simulink model "rsa_simulink"  (R2015a)
settings: Solver=ode45  StartTime=0.0  StopTime=1  RelTol=1e-3
settings Model: Creator=Hp  LastModifiedBy=Hp

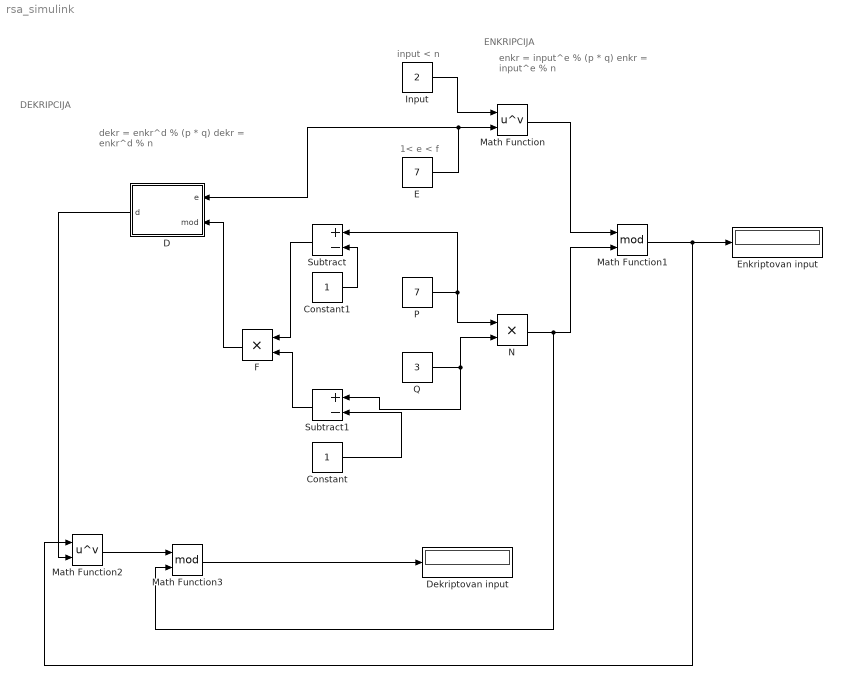
== system rsa_simulink ==
  note: 1< e < f
  note: ENKRIPCIJA
  note: DEKRIPCIJA
  note: enkr = input^e % (p * q)
      | enkr = input^e % n
  note: dekr = enkr^d % (p * q)
      | dekr = enkr^d % n
  note: input < n
  Constant : Constant
  Constant1 : Constant
  D : MATLAB Function  TreatAsAtomicUnit=on
  Dekriptovan input : Display
  E : Constant  Value=7
  Enkriptovan input : Display
  "F " : Product
  Input : Constant  Value=2
  Math Function : Math  Operator=pow  SaturateOnIntegerOverflow=on
  Math Function1 : Math  Operator=mod  SaturateOnIntegerOverflow=on
  Math Function2 : Math  Operator=pow  SaturateOnIntegerOverflow=on
  Math Function3 : Math  Operator=mod  SaturateOnIntegerOverflow=on
  "N " : Product
  P : Constant  Value=7
  Q : Constant  Value=3
  Subtract : Sum  Inputs=+-
  Subtract1 : Sum  Inputs=+-
  wires:
  P/1 -> Subtract/1, "N "/1
  Q/1 -> Subtract1/1, "N "/2
  E/1 -> D/1(e), Math Function/2
  Input/1 -> Math Function/1
  "N "/1 -> Math Function3/2, Math Function1/2
  Math Function/1 -> Math Function1/1
  Constant1/1 -> Subtract/2
  Constant/1 -> Subtract1/2
  Subtract/1 -> "F "/1
  Subtract1/1 -> "F "/2
  "F "/1 -> D/2(mod)
  D/1(d) -> Math Function2/2
  Math Function1/1 -> Math Function2/1, Enkriptovan input/1
  Math Function2/1 -> Math Function3/1
  Math Function3/1 -> Dekriptovan input/1

== matlab function rsa_simulink/D ==
  data: e input; d output; mod input
function d = fcn(e, mod)
%#codegen
d = 1;

% Dok god se ne pronadje broj D koji kada se pomnozi sa e i
% podeli sa mod daje ostatak 1 [POSTOJI OPASNOST OD INF LOOP??]
while(rem((e * d), mod) ~= 1)
    d = d + 1;
end
d = d;
